simulink model "Swarm_Simulation"  (R2019a)
settings: Solver=VariableStepAuto  StartTime=0.0  StopTime=100.0  RelTol=1e-3
values from neighbouring files (symbols this model uses):
  x_ini = 100 * 2 * rand(N,n) - 1    [CMP756_AhmetBurakKOC_HW2.m]    (also in swarm_init.m)
settings Model: Creator=kocab  LastModifiedBy=kocab

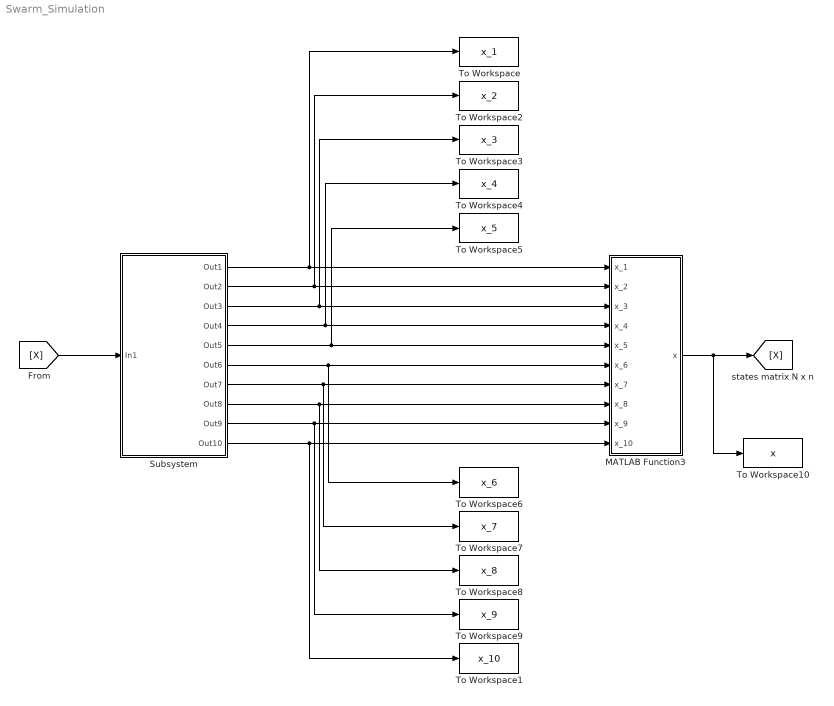
== system Swarm_Simulation ==
  MATLAB Function3 : MATLAB Function  TreatAsAtomicUnit=on
  Subsystem : Subsystem
  To Workspace : ToWorkspace  VariableName=x_1  SampleTime=-1
  To Workspace1 : ToWorkspace  VariableName=x_10  SampleTime=-1
  To Workspace10 : ToWorkspace  VariableName=x  SampleTime=-1
  To Workspace2 : ToWorkspace  VariableName=x_2  SampleTime=-1
  To Workspace3 : ToWorkspace  VariableName=x_3  SampleTime=-1
  To Workspace4 : ToWorkspace  VariableName=x_4  SampleTime=-1
  To Workspace5 : ToWorkspace  VariableName=x_5  SampleTime=-1
  To Workspace6 : ToWorkspace  VariableName=x_6  SampleTime=-1
  To Workspace7 : ToWorkspace  VariableName=x_7  SampleTime=-1
  To Workspace8 : ToWorkspace  VariableName=x_8  SampleTime=-1
  To Workspace9 : ToWorkspace  VariableName=x_9  SampleTime=-1
  wires:
  Subsystem/3(Out3) -> To Workspace3/1, MATLAB Function3/3(x_3)
  [X] -> Subsystem/1(In1)
  Subsystem/7(Out7) -> MATLAB Function3/7(x_7), To Workspace7/1
  Subsystem/4(Out4) -> MATLAB Function3/4(x_4), To Workspace4/1
  Subsystem/9(Out9) -> MATLAB Function3/9(x_9), To Workspace9/1
  Subsystem/10(Out10) -> To Workspace1/1, MATLAB Function3/10(x_10)
  Subsystem/5(Out5) -> MATLAB Function3/5(x_5), To Workspace5/1
  Subsystem/2(Out2) -> To Workspace2/1, MATLAB Function3/2(x_2)
  Subsystem/1(Out1) -> To Workspace/1, MATLAB Function3/1(x_1)
  Subsystem/6(Out6) -> To Workspace6/1, MATLAB Function3/6(x_6)
  Subsystem/8(Out8) -> To Workspace8/1, MATLAB Function3/8(x_8)
  MATLAB Function3/1(x) -> To Workspace10/1, [X]

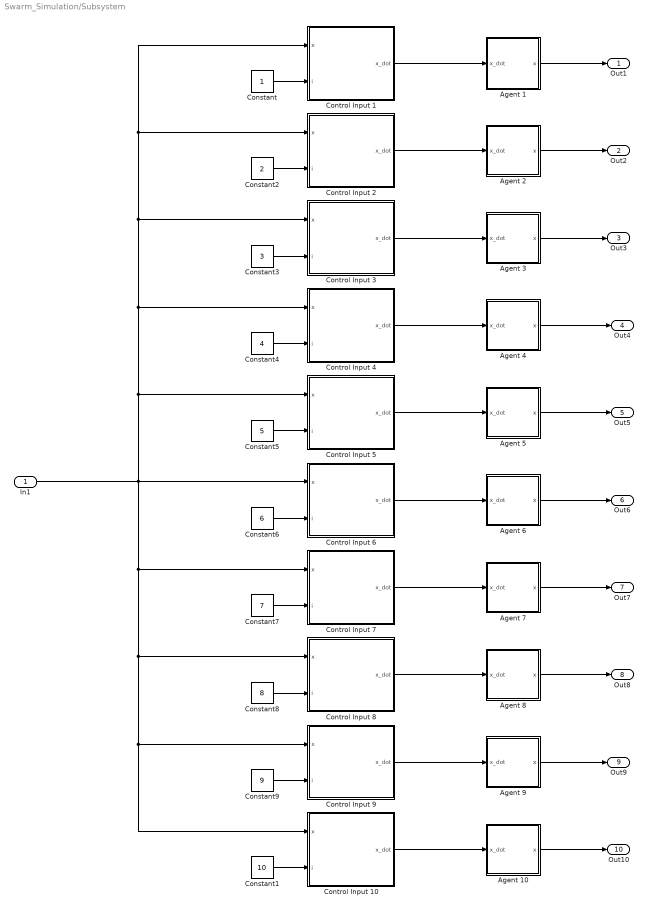
== system Swarm_Simulation/Subsystem ==
  In1 : Inport
  Agent 1 : Subsystem
  Agent 10 : Subsystem
  Agent 2 : Subsystem
  Agent 3 : Subsystem
  Agent 4 : Subsystem
  Agent 5 : Subsystem
  Agent 6 : Subsystem
  Agent 7 : Subsystem
  Agent 8 : Subsystem
  Agent 9 : Subsystem
  Constant : Constant
  Constant1 : Constant  Value=10
  Constant2 : Constant  Value=2
  Constant3 : Constant  Value=3
  Constant4 : Constant  Value=4
  Constant5 : Constant  Value=5
  Constant6 : Constant  Value=6
  Constant7 : Constant  Value=7
  Constant8 : Constant  Value=8
  Constant9 : Constant  Value=9
  Control Input 1 : MATLAB Function  TreatAsAtomicUnit=on
  Control Input 10 : MATLAB Function  TreatAsAtomicUnit=on
  Control Input 2 : MATLAB Function  TreatAsAtomicUnit=on
  Control Input 3 : MATLAB Function  TreatAsAtomicUnit=on
  Control Input 4 : MATLAB Function  TreatAsAtomicUnit=on
  Control Input 5 : MATLAB Function  TreatAsAtomicUnit=on
  Control Input 6 : MATLAB Function  TreatAsAtomicUnit=on
  Control Input 7 : MATLAB Function  TreatAsAtomicUnit=on
  Control Input 8 : MATLAB Function  TreatAsAtomicUnit=on
  Control Input 9 : MATLAB Function  TreatAsAtomicUnit=on
  Out1 : Outport
  Out2 : Outport  Port=2
  Out3 : Outport  Port=3
  Out4 : Outport  Port=4
  Out5 : Outport  Port=5
  Out6 : Outport  Port=6
  Out7 : Outport  Port=7
  Out8 : Outport  Port=8
  Out9 : Outport  Port=9
  Out10 : Outport  Port=10
  wires:
  Constant9/1 -> Control Input 9/2(i)
  Control Input 7/1(x_dot) -> Agent 7/1(x_dot)
  Control Input 9/1(x_dot) -> Agent 9/1(x_dot)
  Constant7/1 -> Control Input 7/2(i)
  Agent 8/1(x) -> Out8/1
  Constant6/1 -> Control Input 6/2(i)
  Constant8/1 -> Control Input 8/2(i)
  Constant3/1 -> Control Input 3/2(i)
  Agent 3/1(x) -> Out3/1
  In1/1 -> Control Input 9/1(x), Control Input 10/1(x), Control Input 8/1(x), Control Input 7/1(x), Control Input 6/1(x), Control Input 5/1(x), Control Input 4/1(x), Control Input 3/1(x), Control Input 2/1(x), Control Input 1/1(x)
  Control Input 6/1(x_dot) -> Agent 6/1(x_dot)
  Control Input 8/1(x_dot) -> Agent 8/1(x_dot)
  Control Input 4/1(x_dot) -> Agent 4/1(x_dot)
  Agent 2/1(x) -> Out2/1
  Constant4/1 -> Control Input 4/2(i)
  Agent 6/1(x) -> Out6/1
  Control Input 10/1(x_dot) -> Agent 10/1(x_dot)
  Constant/1 -> Control Input 1/2(i)
  Constant1/1 -> Control Input 10/2(i)
  Control Input 5/1(x_dot) -> Agent 5/1(x_dot)
  Constant5/1 -> Control Input 5/2(i)
  Control Input 3/1(x_dot) -> Agent 3/1(x_dot)
  Control Input 2/1(x_dot) -> Agent 2/1(x_dot)
  Agent 1/1(x) -> Out1/1
  Agent 5/1(x) -> Out5/1
  Constant2/1 -> Control Input 2/2(i)
  Control Input 1/1(x_dot) -> Agent 1/1(x_dot)
  Agent 7/1(x) -> Out7/1
  Agent 10/1(x) -> Out10/1
  Agent 9/1(x) -> Out9/1
  Agent 4/1(x) -> Out4/1

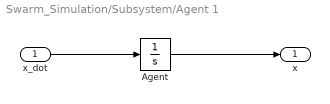
== system Swarm_Simulation/Subsystem/Agent 1 ==
  x_dot : Inport
  Agent : Integrator  InitialCondition=x_ini(1,:)
  x : Outport
  wires:
  x_dot/1 -> Agent/1
  Agent/1 -> x/1

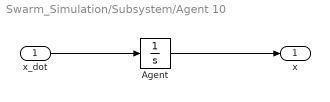
== system Swarm_Simulation/Subsystem/Agent 10 ==
  x_dot : Inport
  Agent : Integrator  InitialCondition=x_ini(10,:)
  x : Outport
  wires:
  x_dot/1 -> Agent/1
  Agent/1 -> x/1

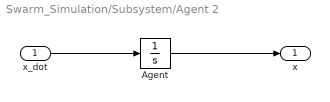
== system Swarm_Simulation/Subsystem/Agent 2 ==
  x_dot : Inport
  Agent : Integrator  InitialCondition=x_ini(2,:)
  x : Outport
  wires:
  x_dot/1 -> Agent/1
  Agent/1 -> x/1

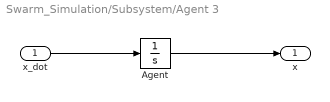
== system Swarm_Simulation/Subsystem/Agent 3 ==
  x_dot : Inport
  Agent : Integrator  InitialCondition=x_ini(3,:)
  x : Outport
  wires:
  x_dot/1 -> Agent/1
  Agent/1 -> x/1

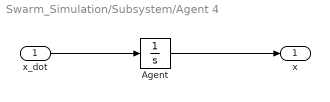
== system Swarm_Simulation/Subsystem/Agent 4 ==
  x_dot : Inport
  Agent : Integrator  InitialCondition=x_ini(4,:)
  x : Outport
  wires:
  x_dot/1 -> Agent/1
  Agent/1 -> x/1

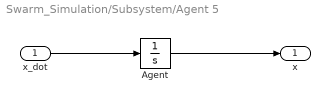
== system Swarm_Simulation/Subsystem/Agent 5 ==
  x_dot : Inport
  Agent : Integrator  InitialCondition=x_ini(5,:)
  x : Outport
  wires:
  x_dot/1 -> Agent/1
  Agent/1 -> x/1

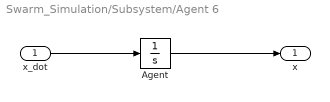
== system Swarm_Simulation/Subsystem/Agent 6 ==
  x_dot : Inport
  Agent : Integrator  InitialCondition=x_ini(6,:)
  x : Outport
  wires:
  x_dot/1 -> Agent/1
  Agent/1 -> x/1

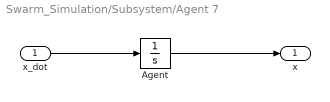
== system Swarm_Simulation/Subsystem/Agent 7 ==
  x_dot : Inport
  Agent : Integrator  InitialCondition=x_ini(7,:)
  x : Outport
  wires:
  x_dot/1 -> Agent/1
  Agent/1 -> x/1

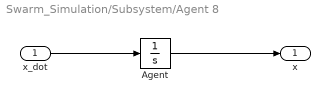
== system Swarm_Simulation/Subsystem/Agent 8 ==
  x_dot : Inport
  Agent : Integrator  InitialCondition=x_ini(8,:)
  x : Outport
  wires:
  x_dot/1 -> Agent/1
  Agent/1 -> x/1

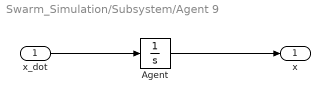
== system Swarm_Simulation/Subsystem/Agent 9 ==
  x_dot : Inport
  Agent : Integrator  InitialCondition=x_ini(9,:)
  x : Outport
  wires:
  x_dot/1 -> Agent/1
  Agent/1 -> x/1

== matlab function Swarm_Simulation/Subsystem/Control Input 10 ==
  data: x input; x_dot output; i input
function x_dot  = control_input(x,i)
x_dot = control_input(x,i);

== matlab function Swarm_Simulation/Subsystem/Control Input 1 ==
  data: x input; x_dot output; i input
function x_dot  = control_input(x,i)
x_dot = control_input(x,i);

== matlab function Swarm_Simulation/Subsystem/Control Input 2 ==
  data: x input; x_dot output; i input
function x_dot  = control_input(x,i)
x_dot = control_input(x,i);

== matlab function Swarm_Simulation/MATLAB Function3 ==
  data: x_1 input; x output; x_2 input; x_3 input; x_4 input; x_5 input; x_6 input; x_7 input; x_8 input; x_9 input; x_10 input
function x = fcn(x_1,x_2,x_3,x_4,x_5,x_6,x_7,x_8,x_9,x_10)
x = [x_1' ; x_2' ; x_3'; x_4'; x_5'; x_6'; x_7'; x_8'; x_9'; x_10'];
end

== matlab function Swarm_Simulation/Subsystem/Control Input 3 ==
  data: x input; x_dot output; i input
function x_dot  = control_input(x,i)
x_dot = control_input(x,i);

== matlab function Swarm_Simulation/Subsystem/Control Input 4 ==
  data: x input; x_dot output; i input
function x_dot  = control_input(x,i)
x_dot = control_input(x,i);

== matlab function Swarm_Simulation/Subsystem/Control Input 5 ==
  data: x input; x_dot output; i input
function x_dot  = control_input(x,i)
x_dot = control_input(x,i);

== matlab function Swarm_Simulation/Subsystem/Control Input 6 ==
  data: x input; x_dot output; i input
function x_dot  = control_input(x,i)
x_dot = control_input(x,i);

== matlab function Swarm_Simulation/Subsystem/Control Input 7 ==
  data: x input; x_dot output; i input
function x_dot  = control_input(x,i)
x_dot = control_input(x,i);

== matlab function Swarm_Simulation/Subsystem/Control Input 8 ==
  data: x input; x_dot output; i input
function x_dot  = control_input(x,i)
x_dot = control_input(x,i);

== matlab function Swarm_Simulation/Subsystem/Control Input 9 ==
  data: x input; x_dot output; i input
function x_dot  = control_input(x,i)
x_dot = control_input(x,i);
